simulink model "vehicleModelBodyAndTires"  (R2024b)
settings: Solver=VariableStepAuto  StartTime=0.0  StopTime=1200  MaxStep=0.1  RelTol=1e-3  AbsTol=1e-3
PreLoadFcn:
  | setVehicleParam
undefined symbols (not defined in the file): wheelInertia
libraries: sdl_lib x6, fl_lib x6, nesl_utility x3
settings Model: Creator=lnicolet  LastModifiedBy=lnicolet
settings SolverCC: AutoScaleAbsTol=off  AlgebraicLoopSolver=TrustRegion  MaxZcPerStep=1
settings DebuggingCC: UnconnectedInputMsg=warning  UnconnectedOutputMsg=warning  UnconnectedLineMsg=warning  SymbolicDimsDataTypeCodeGenerationDiagnostic=none
settings ModelReferenceCC: EnableRefExpFcnMdlSchedulingChecks=on
settings SFSimCC: CustomCodeUndefinedFunction=UseInterfaceOnly
settings RTWCC: GPUComputeCapability=3.5  DLArmComputeVersion=19.05
settings SimscapeCC: SimscapeLogType=all  SimscapeLogSimulationStatistics=on  SimscapeLogLimitData=off  SimscapeLogDataHistory=10000

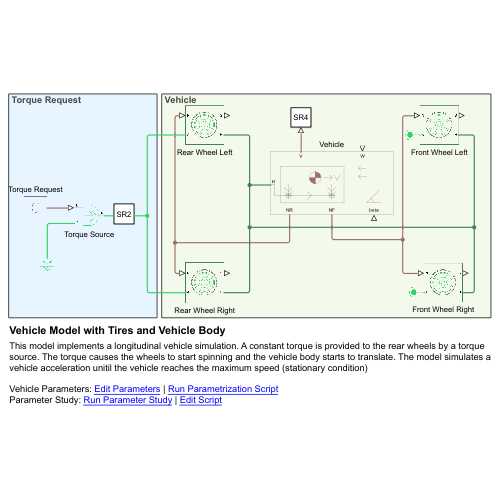
[thumbnail: Simulink's stored preview of the top-level diagram]
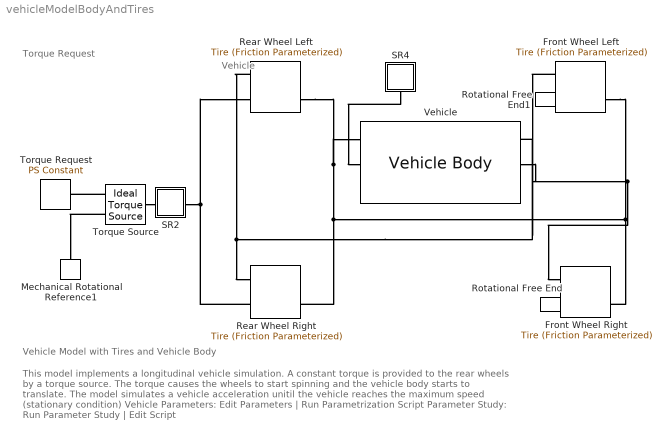
== system vehicleModelBodyAndTires ==
  note: Vehicle
  note: Torque Request
  note: This model implements a longitudinal vehicle simulation. A constant torque is provided to the rear wheels by a torque source. The torque causes the wheels to start spinning and the vehicle body starts to translate. The model simulates a vehicle acceleration unitil the vehicle reaches the maximum speed (stationary condition)
      |
      | Vehicle Parameters: Edit Parameters | Run Parametrization Script
      | Parameter Study: Run Parameter Study | Edit Script
  note: Vehicle Model with Tires and Vehicle Body
  Front Wheel Left : sdl_lib/Tires & Vehicles/Tire (Friction Parameterized)  r_tire=wheelRadius m  slip_output=sdl.enum.SlipOutput.Relative  friction_model=sdl.enum.friction_model_var.fixed  mu_static=0.90  mu_kinetic=0.70  slip_vector=[-1, .6, .15, .06, .02, 0] rad/s  mu_kinetic_vector=[.7, .7, .75, .8, .88, .89]  interp_method=simscape.enum.interpolation.linear  extrap_method=simscape.enum.extrapolation.linear  model_compliance=sdl.enum.compliance.off  stiffness=1e6 N/m  damping=1000 N*s/m  model_inertia=true  wheel_inertia=wheelInertia(1) kg*m^2  belt_inertia=wheelInertia(2) kg*m^2  initial_velocity=wheelSpeedStart rad/s  model_resistance=simscape.enum.onoff.on  resistance_model=sdl.enum.RollingResistance.Constant  coeff=0.015  p_tire=250e3 Pa  alpha=-0.003  beta=0.97  coeff_a=84e-4  coeff_b=6.2e-4 s/m  coeff_c=1.6e-4 s^2/m^2  v_thr=0.001 m/s  v_tol=0.001 m/s  F_min=10 N  initial_traction_state=sdl.enum.tireIC.slipping
      settings: InternalSimscapePortConfiguration="{\"Bottom\":[],\"Left\":[{\"id\":\"N\",\"label\":\"N\",\"type\":\"input\"},{\"id\":\"A\",\"label\":\"A\",\"type\":\"foundation.mechanical.rotational.rotational\"}],\"Right\":[{\"id\":\"Srel\",\"label\":\"S\",\"type\":\"output\"},{\"id\":\"H\",\"label\":\"H\",\"type\":\"foundation.mechanical.translational.translational\"}],\"Top\":[]}"
  Front Wheel Right : sdl_lib/Tires & Vehicles/Tire (Friction Parameterized)  r_tire=wheelRadius m  slip_output=sdl.enum.SlipOutput.Relative  friction_model=sdl.enum.friction_model_var.fixed  mu_static=0.90  mu_kinetic=0.70  slip_vector=[-1, .6, .15, .06, .02, 0] rad/s  mu_kinetic_vector=[.7, .7, .75, .8, .88, .89]  interp_method=simscape.enum.interpolation.linear  extrap_method=simscape.enum.extrapolation.linear  model_compliance=sdl.enum.compliance.off  stiffness=1e6 N/m  damping=1000 N*s/m  model_inertia=true  wheel_inertia=wheelInertia(1) kg*m^2  belt_inertia=wheelInertia(2) kg*m^2  initial_velocity=wheelSpeedStart rad/s  model_resistance=simscape.enum.onoff.on  resistance_model=sdl.enum.RollingResistance.Constant  coeff=0.015  p_tire=250e3 Pa  alpha=-0.003  beta=0.97  coeff_a=84e-4  coeff_b=6.2e-4 s/m  coeff_c=1.6e-4 s^2/m^2  v_thr=0.001 m/s  v_tol=0.001 m/s  F_min=10 N  initial_traction_state=sdl.enum.tireIC.slipping
      settings: InternalSimscapePortConfiguration="{\"Bottom\":[],\"Left\":[{\"id\":\"N\",\"label\":\"N\",\"type\":\"input\"},{\"id\":\"A\",\"label\":\"A\",\"type\":\"foundation.mechanical.rotational.rotational\"}],\"Right\":[{\"id\":\"Srel\",\"label\":\"S\",\"type\":\"output\"},{\"id\":\"H\",\"label\":\"H\",\"type\":\"foundation.mechanical.translational.translational\"}],\"Top\":[]}"
  Mechanical Rotational Reference1 : fl_lib/Mechanical/Rotational Elements/Mechanical Rotational Reference
  Rear Wheel Left : sdl_lib/Tires & Vehicles/Tire (Friction Parameterized)  r_tire=wheelRadius m  slip_output=sdl.enum.SlipOutput.Relative  friction_model=sdl.enum.friction_model_var.fixed  mu_static=0.90  mu_kinetic=0.70  slip_vector=[-1, .6, .15, .06, .02, 0] rad/s  mu_kinetic_vector=[.7, .7, .75, .8, .88, .89]  interp_method=simscape.enum.interpolation.linear  extrap_method=simscape.enum.extrapolation.linear  model_compliance=sdl.enum.compliance.off  stiffness=1e6 N/m  damping=1000 N*s/m  model_inertia=true  wheel_inertia=wheelInertia(1) kg*m^2  belt_inertia=wheelInertia(2) kg*m^2  initial_velocity=wheelSpeedStart rad/s  model_resistance=simscape.enum.onoff.on  resistance_model=sdl.enum.RollingResistance.Constant  coeff=0.015  p_tire=250e3 Pa  alpha=-0.003  beta=0.97  coeff_a=84e-4  coeff_b=6.2e-4 s/m  coeff_c=1.6e-4 s^2/m^2  v_thr=0.001 m/s  v_tol=0.001 m/s  F_min=10 N  initial_traction_state=sdl.enum.tireIC.slipping
      settings: InternalSimscapePortConfiguration="{\"Bottom\":[],\"Left\":[{\"id\":\"N\",\"label\":\"N\",\"type\":\"input\"},{\"id\":\"A\",\"label\":\"A\",\"type\":\"foundation.mechanical.rotational.rotational\"}],\"Right\":[{\"id\":\"Srel\",\"label\":\"S\",\"type\":\"output\"},{\"id\":\"H\",\"label\":\"H\",\"type\":\"foundation.mechanical.translational.translational\"}],\"Top\":[]}"
  Rear Wheel Right : sdl_lib/Tires & Vehicles/Tire (Friction Parameterized)  r_tire=wheelRadius m  slip_output=sdl.enum.SlipOutput.Relative  friction_model=sdl.enum.friction_model_var.fixed  mu_static=0.90  mu_kinetic=0.70  slip_vector=[-1, .6, .15, .06, .02, 0] rad/s  mu_kinetic_vector=[.7, .7, .75, .8, .88, .89]  interp_method=simscape.enum.interpolation.linear  extrap_method=simscape.enum.extrapolation.linear  model_compliance=sdl.enum.compliance.off  stiffness=1e6 N/m  damping=1000 N*s/m  model_inertia=true  wheel_inertia=wheelInertia(1) kg*m^2  belt_inertia=wheelInertia(2) kg*m^2  initial_velocity=wheelSpeedStart rad/s  model_resistance=simscape.enum.onoff.on  resistance_model=sdl.enum.RollingResistance.Constant  coeff=0.015  p_tire=250e3 Pa  alpha=-0.003  beta=0.97  coeff_a=84e-4  coeff_b=6.2e-4 s/m  coeff_c=1.6e-4 s^2/m^2  v_thr=0.001 m/s  v_tol=0.001 m/s  F_min=10 N  initial_traction_state=sdl.enum.tireIC.slipping
      settings: InternalSimscapePortConfiguration="{\"Bottom\":[],\"Left\":[{\"id\":\"N\",\"label\":\"N\",\"type\":\"input\"},{\"id\":\"A\",\"label\":\"A\",\"type\":\"foundation.mechanical.rotational.rotational\"}],\"Right\":[{\"id\":\"Srel\",\"label\":\"S\",\"type\":\"output\"},{\"id\":\"H\",\"label\":\"H\",\"type\":\"foundation.mechanical.translational.translational\"}],\"Top\":[]}"
  Rotational Free End : fl_lib/Mechanical/Rotational Elements/Rotational Free End  w_specify=off  w_priority=None  w=0 rad/s  w_nominal_specify=off  w_nominal_value=1  w_nominal_unit=rad/s
  Rotational Free End1 : fl_lib/Mechanical/Rotational Elements/Rotational Free End  w_specify=off  w_priority=None  w=0 rad/s  w_nominal_specify=off  w_nominal_value=1  w_nominal_unit=rad/s
  SR2 : Subsystem
      settings: PortSchema="{\"entries\":[{\"content\":{\"sides\":[{\"content\":{},\"type\":\"ConnectorPlacement.EquallySpacedRectSide\",\"uuid\":\"85a1558c-1b31-403a-adff-1ac0e6328287\"},{\"content\":{\"side\":\"RIGHT\"},\"type\":\"ConnectorPlacement.EquallySpacedRectSide\",\"uuid\":\"de598219-9a5a-4194-bdeb-930f1cdc45c3\"},{\"content\":{\"connectorIds\":[\"LConn1\"],\"side\":\"TOP\"},\"type\":\"ConnectorPlacement.EquallySpacedRectSide\",\"uuid\":\"10bc604a-047d-4d1a-b0b7-1fa83a2f0568\"},{\"content\":{\"connectorIds\":[\"RConn1\"],\"side\":\"BOTTOM\"},\"type\":\"ConnectorPlacement.EquallySpacedRectSide\",\"uuid\":\"148b1bdb-f9c4-471d-a1fa-71cb1ae939b1\"}]},\"type\":\"ConnectorPlacement.EquallySpacedConnector\",\"uuid\":\"121a5661-41e8-4645-ac4e-8b084eb01302\"}],\"packageUris\":[\"http://schema.mathworks.com/mf0/Connector/R2020b\"],\"version\":\"1.0\"}"
      settings: OpenFcn=|
      | scopePath = [gcb '/Scope'];
      | open_system(scopePath);
      mask Display: disp(get_param(gcb,'Name'))
  SR4 : Subsystem
      settings: OpenFcn=|
      | scopePath = [gcb '/Scope'];
      | open_system(scopePath);
      mask Display: disp(get_param(gcb,'Name'));
  Torque Request : fl_lib/Physical Signals/Sources/PS Constant  constant=100 N*m
  Torque Source : fl_lib/Mechanical/Mechanical Sources/Ideal Torque Source
  Vehicle : sdl_lib/Tires & Vehicles/Vehicle Body  mass=vehicleMass kg  n_w=2  x_f=vehicleCOGFA m  x_r=vehicleCOGRA m  y_c=0.5 m  mass_var=false  g=9.81 m/s^2  liftoff_warning=false  area=vehicleSurf m^2  Cd_var=false  Cd=vehicleCD  rho=1.18 kg/m^3  model_pitch=false  inertia=4000 kg*m^2  suspension_model=sdl.enum.linearTLU.linear  k_f=1e4 N/m  b_f=1e4 N*s/m  k_r=1e4 N/m  b_r=1e4 N*s/m  k_f_TLU=[-2000, -1000, 0, 1000, 2000] N  x_f_TLU=[-.4, -.2, 0, .2, .4] m  b_f_TLU=[-200, -100, 0, 100, 200] N  v_f_TLU=[-4, -2, 0, 2, 4] m/s  k_r_TLU=[-2000, -1000, 0, 1000, 2000] N  x_r_TLU=[-.4, -.2, 0, .2, .4] m  b_r_TLU=[-200, -100, 0, 100, 200] N  v_r_TLU=[-4, -2, 0, 2, 4] m/s  interp_method=simscape.enum.interpolation.linear  extrap_method=simscape.enum.extrapolation.linear  model_hardstop=false  upper_bound_f=.25 m  lower_bound_f=-.25 m  stop_k_f=1e6 N/m  stop_b_f=150 N*s/m  upper_bound_r=.25 m  lower_bound_r=-.25 m  stop_k_r=1e6 N/m  stop_b_r=150 N*s/m  initial_pitch=0 rad  initial_pitch_rate=0 rad/s  v_specify=on  v_priority=High  v=0 m/s  v_nominal_specify=off  v_nominal_value=1  v_nominal_unit=m/s
      settings: InternalSimscapePortConfiguration="{\"Bottom\":[{\"id\":\"NR\",\"label\":\"NR\",\"type\":\"output\"},{\"id\":\"NF\",\"label\":\"NF\",\"type\":\"output\"},{\"id\":\"beta\",\"label\":\"beta\",\"type\":\"input\"}],\"Left\":[{\"id\":\"H\",\"label\":\"H\",\"type\":\"foundation.mechanical.translational.translational\"}],\"Right\":[],\"Top\":[{\"id\":\"V\",\"label\":\"V\",\"type\":\"output\"},{\"id\":\"wind\",\"label\":\"W\",\"type\":\"input\"}]}"
  connections:
  Rear Wheel Left/RConn2 -- Rear Wheel Right/RConn2 -- Front Wheel Right/RConn2 -- Front Wheel Left/RConn2 -- Vehicle/LConn1
  Rear Wheel Left/LConn1 -- Rear Wheel Right/LConn1 -- Vehicle/RConn1
  Vehicle/RConn2 -- Front Wheel Left/LConn1 -- Front Wheel Right/LConn1
  SR4/LConn1 -- Vehicle/LConn2
  Rear Wheel Right/LConn2 -- SR2/RConn1 -- Rear Wheel Left/LConn2
  Rotational Free End/LConn1 -- Front Wheel Right/LConn2
  Rotational Free End1/LConn1 -- Front Wheel Left/LConn2
  Torque Source/RConn1 -- Torque Request/RConn1
  Torque Source/RConn2 -- Mechanical Rotational Reference1/LConn1
  Torque Source/LConn1 -- SR2/LConn1

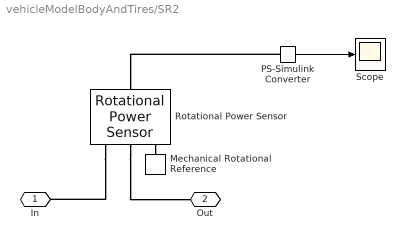
== system vehicleModelBodyAndTires/SR2 ==
  Mechanical Rotational Reference : fl_lib/Mechanical/Rotational Elements/Mechanical Rotational Reference
  PS-Simulink Converter : nesl_utility/PS-Simulink Converter  PhysicalDomain=network_engine_domain  SubClassName=ps_output  LeftPortType=input  RightPortType=output  PseudoPeriodic=off  Frequencies=[]  VectorFormat=inherit  Unit=kW  AffineConversion=off
  Rotational Power Sensor : sdl_lib/Sensors/Rotational Power Sensor  measurement_type=sdl.enum.rotationalPowerSensorType.instantaneous  averaging_period=1 s  max_frequency=1000 Hz  max_speed=1000 rpm
      settings: InternalSimscapePortConfiguration="{\"Bottom\":[],\"Left\":[{\"id\":\"S\",\"label\":\"S\",\"type\":\"foundation.mechanical.rotational.rotational\"},{\"id\":\"R\",\"label\":\"R\",\"type\":\"foundation.mechanical.rotational.rotational\"},{\"id\":\"C\",\"label\":\"C\",\"type\":\"foundation.mechanical.rotational.rotational\"}],\"Right\":[{\"id\":\"P\",\"label\":\"P\",\"type\":\"output\"}],\"Top\":[]}"
  Scope : Scope
  In : PMIOPort  Side=Left
  Out : PMIOPort  Port=2  Side=Right
  wires:
  PS-Simulink Converter/1 -> Scope/1
  connections:
  Rotational Power Sensor/LConn1 -- In/RConn1
  Rotational Power Sensor/LConn2 -- Out/RConn1
  Rotational Power Sensor/LConn3 -- Mechanical Rotational Reference/LConn1
  PS-Simulink Converter/LConn1 -- Rotational Power Sensor/RConn1

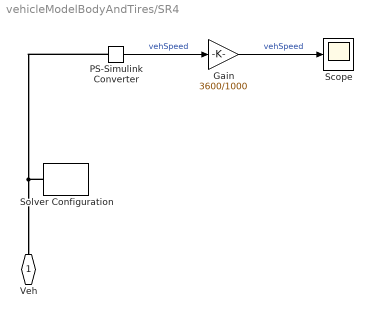
== system vehicleModelBodyAndTires/SR4 ==
  Gain : Gain  Gain=3600/1000
  PS-Simulink Converter : nesl_utility/PS-Simulink Converter  PhysicalDomain=network_engine_domain  SubClassName=ps_output  LeftPortType=input  RightPortType=output  PseudoPeriodic=off  Frequencies=[]  VectorFormat=inherit  Unit=m/s  AffineConversion=off
  Scope : Scope
  Solver Configuration : nesl_utility/Solver Configuration  PhysicalDomain=network_engine_domain  SubClassName=solver  LeftPortType=input  RightPortType=generic  Tones=[]  Harmonics=[]  SimulateNoise=off  Profile=off  UseLocalSampling=off  EnableSwitchedLinearOptims=on  FrequencyDomain=off  UseCCode=off  RelTol=0.001  AbsTol=1e-06  MinStep=1e-09  ToWorkspace=off  RevertToSquareIcSolve=off  NumHomotopyIterations=100  PhasorMode=off  PhasorModeNumHarmonics=1  ConsistencySolver=NEWTON_XTOL_AFTER_FTOL  IndexReductionMethod=DerivativeReplacement  DoDC=off  ResidualTolerance=1e-09  ConsistencyTolSource=GLOBAL  ConsistencyAbsTol=0.001  ConsistencyRelTol=0.001  ConsistencyTolFactor=0.001  UseLocalSolver=off  LocalSolverChoice=NE_BACKWARD_EULER_ADVANCER  ResolveIndetEquations=on  FunctionEvalNumThread=1  LocalSolverSampleTime=0.001  DoFixedCost=off  MaxNonlinIter=3  MaxModeIter=2  ComputeImpulses=off  ImpulseIterations=2  LinearAlgebra=auto  LinearAlgebraNumThread=0  EquationFormulation=NE_TIME_EF  DelaysMemoryBudget=1024  AutomaticFiltering=on  FilteringTimeConstant=0.001  PartitionStorageMethod=AS_NEEDED  PartitionMemoryBudget=1024  PartitionMethod=ROBUST  MultibodyUseLocalSolver=off  MultibodyLocalSolverChoice=ODE1  MultibodyLocalSolverSampleTime=0.001
  Veh : PMIOPort  Side=Left
  wires:
  PS-Simulink Converter/1 -> Gain/1  "vehSpeed"
  Gain/1 -> Scope/1  "vehSpeed"
  connections:
  PS-Simulink Converter/LConn1 -- Veh/RConn1 -- Solver Configuration/RConn1
